simulink model "model_3_optimum"  (R2022a)
settings: Solver=VariableStepAuto  StartTime=0.0  StopTime=30  RelTol=1e-3
values from neighbouring files (symbols this model uses):
  A = [6, 7, -4, 8; 0, 9, 0, 15; 10, 13, -6, 19; 0, -6, 0, -9]    [task_2.m]
  C = eye(4)    [task_2.m]
  x0 = [1; -1; 1; -1]    [task_2.m]
undefined symbols (not defined in the file or in its folder): L, x_0
settings Model: Creator=vital  LastModifiedBy=Family
settings DebuggingCC: UnconnectedInputMsg=warning  UnconnectedOutputMsg=warning  UnconnectedLineMsg=warning
settings RTWCC: DLArmComputeVersion=19.05

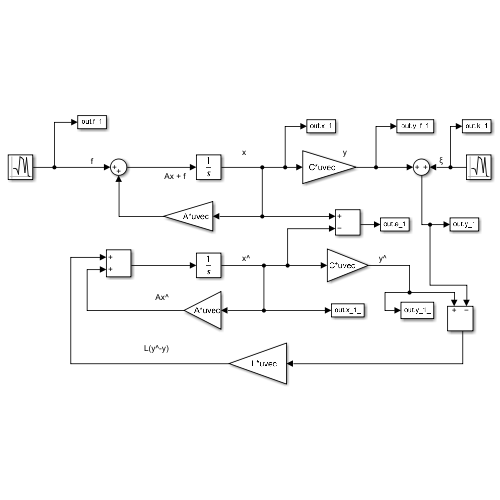
[thumbnail: Simulink's stored preview of the top-level diagram]
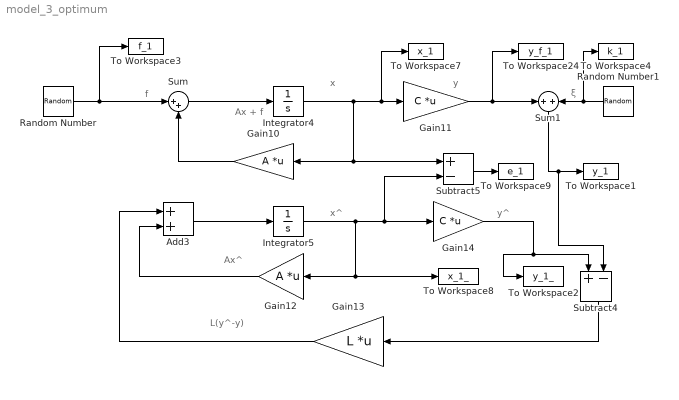
== system model_3_optimum ==
  note: ξ
  note: f
  note: y
  note: Ax^
  note: Ax + f
  note: x
  note: y^
  note: x^
  note: L(y^-y)
  Add3 : Sum
  Gain10 : Gain  Gain=A  Multiplication=Matrix(K*u) (u vector)
  Gain11 : Gain  Gain=C  Multiplication=Matrix(K*u) (u vector)
  Gain12 : Gain  Gain=A  Multiplication=Matrix(K*u) (u vector)
  Gain13 : Gain  Gain=L  Multiplication=Matrix(K*u) (u vector)
  Gain14 : Gain  Gain=C  Multiplication=Matrix(K*u) (u vector)
  Integrator4 : Integrator  InitialCondition=x0
  Integrator5 : Integrator  InitialCondition=x_0
  Random Number : RandomNumber  Variance=65  Seed=[1; 2; 3; 4]  SampleTime=0000.1
  Random Number1 : RandomNumber  Variance=80  Seed=[5 ; 6]  SampleTime=00000.1
  Subtract4 : Sum  Inputs=+-
  Subtract5 : Sum  Inputs=+-
  Sum : Sum  Inputs=|++
  Sum1 : Sum  Inputs=+|+
  To Workspace1 : ToWorkspace  VariableName=y_1  SaveFormat=Timeseries  SampleTime=-1
  To Workspace2 : ToWorkspace  VariableName=y_1_  SaveFormat=Timeseries  SampleTime=-1
  To Workspace24 : ToWorkspace  VariableName=y_f_1  SaveFormat=Timeseries  SampleTime=-1
  To Workspace3 : ToWorkspace  VariableName=f_1  SaveFormat=Timeseries  SampleTime=-1
  To Workspace4 : ToWorkspace  VariableName=k_1  SaveFormat=Timeseries  SampleTime=-1
  To Workspace7 : ToWorkspace  VariableName=x_1  SaveFormat=Timeseries  SampleTime=0.00001
  To Workspace8 : ToWorkspace  VariableName=x_1_  SaveFormat=Timeseries  SampleTime=-1
  To Workspace9 : ToWorkspace  VariableName=e_1  SaveFormat=Timeseries  SampleTime=-1
  wires:
  Gain10/1 -> Sum/2
  Integrator4/1 -> Gain10/1, Subtract5/1, To Workspace7/1, Gain11/1
  Integrator5/1 -> To Workspace8/1, Gain12/1, Subtract5/2, Gain14/1
  Add3/1 -> Integrator5/1
  Gain14/1 -> Subtract4/1, To Workspace2/1
  Gain12/1 -> Add3/2
  Subtract4/1 -> Gain13/1
  Gain13/1 -> Add3/1
  Subtract5/1 -> To Workspace9/1
  Random Number/1 -> Sum/1, To Workspace3/1
  Sum/1 -> Integrator4/1
  Sum1/1 -> Subtract4/2, To Workspace1/1
  Random Number1/1 -> Sum1/2, To Workspace4/1
  Gain11/1 -> To Workspace24/1, Sum1/1
